simulink model "step_01_speed_measurement"  (R2021b)
settings: Solver=FixedStepAuto  StartTime=0.0  StopTime=1.5  FixedStep=1e-6  RelTol=1e-3
model workspace (MATLAB code in the model file):
  | %% DC motor parameteres
  | % High power w/ carbon brushes [3075]
  | % https://github.com/kpierzynski/MiniEmpathiaBot/blob/master/datasheets/POLOLU_N20_MOTOR.pdf
  | Vn = 6;          % [V]
  | Te_stall = 16;   % [kg*mm]
  | S_no_load = 330; % [rpm]
  | N_gear = 100.37; % [-]
  | 
  | La = 1e-4;       % [H]       -> ???
  | J = 1e-7;        % [kg*m^2]  -> ???
  | 
  | %% Incremental encoder parameteres
  | p_enc = 12;  % [pulses per revolution]
  | V_enc = 3.3; % [V]
  | 
  | %% Speed measurement algorithm parameteres
  | % method M sample time
  | Ts = 1e-3; % [s]
  | % Low-pass filter
  | % TODO
libraries: fl_lib x8, nesl_utility x7, spsEdgeDetectorLib x3, ee_lib x2, cstblocks x1, eeGeneralControl x1
settings Model: Creator=adria  LastModifiedBy=adria

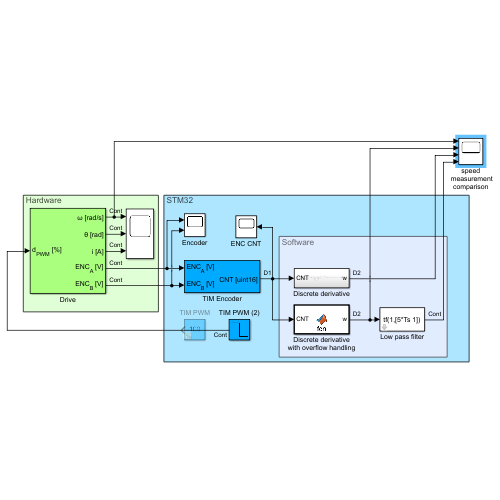
[thumbnail: Simulink's stored preview of the top-level diagram]
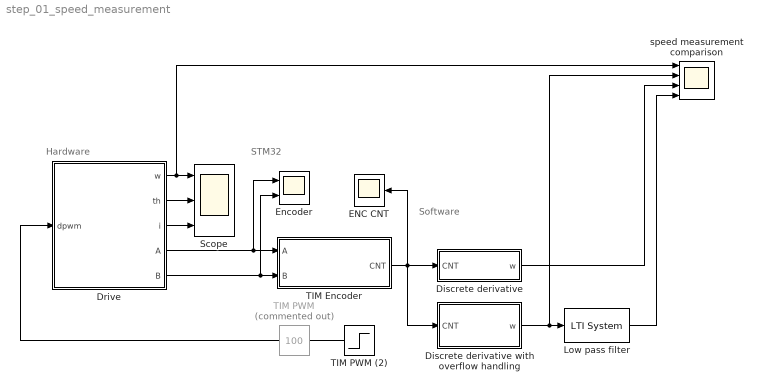
== system step_01_speed_measurement ==
  note: Software
  note: STM32
  note: Hardware
  Discrete derivative : Subsystem
  Discrete derivative with overflow handling : MATLAB Function  TreatAsAtomicUnit=on
  Drive : Subsystem
      mask Display:
      | port_label('input',1,'d_{PWM} [%]','texmode','on');
      | port_label('output',1,'\omega [rad/s]','texmode','on');
      | port_label('output',2,'\theta [rad]','texmode','on');
      | port_label('output',3,'i [A]','texmode','on');
      | port_label('output',4,'ENC_A [V]','texmode','on');
      | port_label('output',5,'ENC_B [V]','texmode','on');
  ENC CNT : Scope
  Encoder : Scope  NumInputPorts=2
  Low pass filter : cstblocks/LTI System  sys=tf(1,[5*Ts 1])  IC=[]
  Scope : Scope  NumInputPorts=3
  TIM Encoder : Subsystem
      mask Display:
      | port_label('input',1','ENC_A [V]','texmode','on');
      | port_label('input',2','ENC_B [V]','texmode','on');
      | port_label('output',1','CNT [uint16]','texmode','on');
  TIM PWM : Constant  Commented=on  Value=100
  TIM PWM (2) : Step  Time=0.5  Before=100  After=-100  SampleTime=0
  speed measurement comparison : Scope  NumInputPorts=4
  wires:
  TIM PWM (2)/1 -> Drive/1(dpwm)
  Drive/1(w) -> speed measurement comparison/1, Scope/1
  Drive/2(th) -> Scope/2
  Drive/3(i) -> Scope/3
  Drive/4(A) -> TIM Encoder/1(A), Encoder/1
  Drive/5(B) -> Encoder/2, TIM Encoder/2(B)
  TIM Encoder/1(CNT) -> Discrete derivative with overflow handling/1(CNT), Discrete derivative/1(CNT), ENC CNT/1
  Discrete derivative with overflow handling/1(w) -> speed measurement comparison/2, Low pass filter/1
  Low pass filter/1 -> speed measurement comparison/4
  Discrete derivative/1(w) -> speed measurement comparison/3

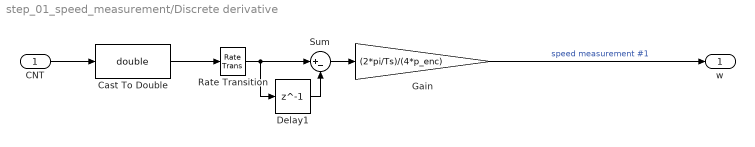
== system step_01_speed_measurement/Discrete derivative ==
  CNT : Inport
  Cast To Double : DataTypeConversion  OutDataTypeStr=double
  Delay1 : Delay  DelayLength=1  InitialCondition=60000  SampleTime=Ts
  Gain : Gain  Gain=(2*pi/Ts)/(4*p_enc)
  Rate Transition : RateTransition  OutPortSampleTime=Ts
  Sum : Sum  Inputs=|+-
  w : Outport  Unit=rad/s
  wires:
  Gain/1 -> w/1  "speed measurement #1"
  CNT/1 -> Cast To Double/1
  Sum/1 -> Gain/1
  Delay1/1 -> Sum/2
  Rate Transition/1 -> Delay1/1, Sum/1
  Cast To Double/1 -> Rate Transition/1

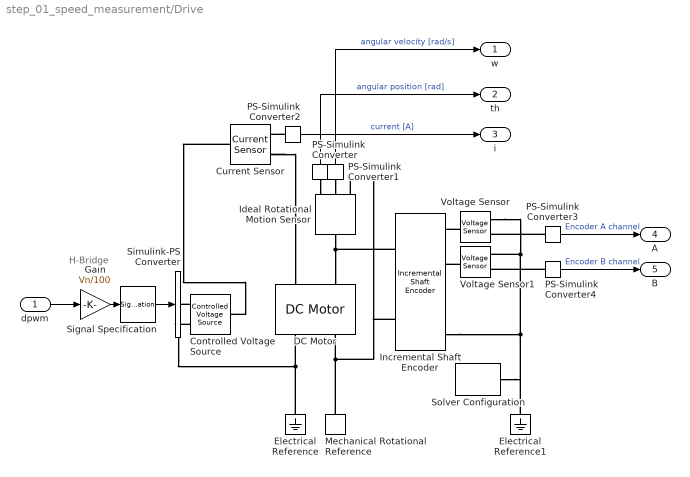
== system step_01_speed_measurement/Drive ==
  note: H-Bridge
  dpwm : Inport  Unit=1
  Controlled Voltage Source : fl_lib/Electrical/Electrical Sources/Controlled Voltage Source
  Current Sensor : fl_lib/Electrical/Electrical Sensors/Current Sensor
  DC Motor : ee_lib/Electromechanical/Brushed Motors/DC Motor  field_option=ee.enum.field_option.pm  Rf=100 Ohm  Lf=1 H  Laf=0.15 H  If0=0 A  parameterization=ee.enum.dcparam_option.torque_speed  Ra=Ra Ohm  La=La H  emf_or_torque=ee.enum.emf_or_torque.kv  Kv=2e-3 V/(rad/s)  Ki=6.876e-4 N*m/A  T_stall=Te_stall mN*m  w_max=S_no_load*N_gear rpm  w_rated=15000 rpm  P_rated=0.08 W  V_rated=Vn V  lam_param=ee.enum.lam_param.damping  i_noload=0 A  V_i_noload=1.5 V  J=J kg*m^2  lam=0 N*m/(rad/s)  speed0=0 rpm  enable_fault_armature=simscape.enum.onoff.off  rev_faulted=1 / 3  G_faulted_armature=1e-5 S  fault_trigger_armature=ee.enum.faults.faultTrigger.temporal  t_fault_armature=1 s  max_permissible_current_armature=inf A  t_fail_on_current_armature=1 s  enable_fault_field=simscape.enum.onoff.off  G_faulted_field=1e-5 S  fault_trigger_field=ee.enum.faults.faultTrigger.temporal  t_fault_field=1 s  max_permissible_current_field=inf A  t_fail_on_current_field=1 s  fault_action=simscape.enum.assert.action.none  alpha=3.93e-3 1/K  Tmeas=25 degC  thermal_mass=100 J/K  initial_temperature=25 degC
  Electrical Reference : fl_lib/Electrical/Electrical Elements/Electrical Reference
  Electrical Reference1 : fl_lib/Electrical/Electrical Elements/Electrical Reference
  Gain : Gain  Gain=Vn/100
  Ideal Rotational Motion Sensor : fl_lib/Mechanical/Mechanical Sensors/Ideal Rotational Motion Sensor  wrap_angle=simscape.enum.onoff.on  offset=0 rad
  Incremental Shaft Encoder : ee_lib/Sensors & Transducers/Incremental Shaft Encoder  NPulse=p_enc  Vm=V_enc V  angle0=0 deg
      settings: SourceProductBaseCode=PS  InternalSimscapePortConfiguration="{\"Bottom\":[],\"Left\":[{\"id\":\"R\",\"label\":\"R\",\"type\":\"foundation.mechanical.rotational.rotational\"},{\"id\":\"C\",\"label\":\"C\",\"type\":\"foundation.mechanical.rotational.rotational\"}],\"Right\":[{\"id\":\"A\",\"label\":\"A\",\"type\":\"foundation.electrical.electrical\"},{\"id\":\"B\",\"label\":\"B\",\"type\":\"foundation.electrical.electrical\"},{\"id\":\"Z\",\"label\":\"Z\",\"type\":\"foundation.electrical.electrical\"},{\"id\":\"GND\",\"label\":\"REF\",\"type\":\"foundation.electrical.electrical\"}],\"Top\":[]}"
  Mechanical Rotational Reference : fl_lib/Mechanical/Rotational Elements/Mechanical Rotational Reference
  PS-Simulink Converter{,1..4} (5 alike) : nesl_utility/PS-Simulink Converter  PhysicalDomain=network_engine_domain  SubClassName=ps_output  LeftPortType=input  RightPortType=output  PseudoPeriodic=off  Frequencies=[]  Unit=inherit  AffineConversion=off
      settings: SourceProductBaseCode=PW,SS
  Signal Specification : SignalSpecification  Unit=V
  Simulink-PS Converter : nesl_utility/Simulink-PS Converter  PhysicalDomain=network_engine_domain  SubClassName=ps_input  LeftPortType=input  RightPortType=output  PseudoPeriodic=off  Frequencies=[]  NoiseDistribution=none  NoiseParameters=[]  Unit=V  AffineConversion=off  FilteringAndDerivatives=provide  SimscapeFilterOrder=1  InputFilterTimeConstant=0.001  UdotUserProvided=0
      settings: SourceProductBaseCode=PW,SS
  Solver Configuration : nesl_utility/Solver Configuration  PhysicalDomain=network_engine_domain  SubClassName=solver  LeftPortType=input  RightPortType=generic  Tones=[]  Harmonics=[]  SimulateNoise=off  Profile=off  UseLocalSampling=off  EnableSwitchedLinearOptims=on  FrequencyDomain=off  UseCCode=off  RelTol=0.001  AbsTol=1e-06  MinStep=1e-09  ToWorkspace=off  RevertToSquareIcSolve=off  NumHomotopyIterations=100  PhasorMode=off  PhasorModeNumHarmonics=1  DoDC=off  ResidualTolerance=1e-09  UseLocalSolver=off  LocalSolverChoice=NE_BACKWARD_EULER_ADVANCER  LocalSolverSampleTime=0.001  DoFixedCost=off  MaxNonlinIter=3  MaxModeIter=2  ComputeImpulses=off  ImpulseIterations=2  LinearAlgebra=auto  EquationFormulation=NE_TIME_EF  DelaysMemoryBudget=1024  AutomaticFiltering=on  FilteringTimeConstant=0.001  PartitionStorageMethod=AS_NEEDED  PartitionMemoryBudget=1024  PartitionMethod=ROBUST
      settings: SourceProductBaseCode=PW,SS
  Voltage Sensor : fl_lib/Electrical/Electrical Sensors/Voltage Sensor
  Voltage Sensor1 : fl_lib/Electrical/Electrical Sensors/Voltage Sensor
  w : Outport  Unit=rad/s
  th : Outport  Port=2  Unit=rad
  i : Outport  Port=3  Unit=A
  A : Outport  Port=4  Unit=V
  B : Outport  Port=5  Unit=V
  wires:
  PS-Simulink Converter2/1 -> i/1  "current [A]"
  PS-Simulink Converter/1 -> th/1  "angular position [rad]"
  PS-Simulink Converter3/1 -> A/1  "Encoder A channel"
  dpwm/1 -> Gain/1
  PS-Simulink Converter4/1 -> B/1  "Encoder B channel"
  PS-Simulink Converter1/1 -> w/1  "angular velocity [rad/s]"
  Gain/1 -> Signal Specification/1
  Signal Specification/1 -> Simulink-PS Converter/1
  connections:
  Ideal Rotational Motion Sensor/RConn1 -- Incremental Shaft Encoder/LConn2 -- DC Motor/RConn2 -- Mechanical Rotational Reference/LConn1
  Controlled Voltage Source/RConn2 -- DC Motor/RConn1 -- Electrical Reference/LConn1
  Solver Configuration/RConn1 -- Electrical Reference1/LConn1 -- Incremental Shaft Encoder/RConn4 -- Voltage Sensor/RConn2 -- Voltage Sensor1/RConn2
  Incremental Shaft Encoder/LConn1 -- DC Motor/LConn2 -- Ideal Rotational Motion Sensor/LConn1
  Voltage Sensor/LConn1 -- Incremental Shaft Encoder/RConn1
  PS-Simulink Converter3/LConn1 -- Voltage Sensor/RConn1
  Voltage Sensor1/LConn1 -- Incremental Shaft Encoder/RConn2
  Current Sensor/LConn1 -- Controlled Voltage Source/LConn1
  PS-Simulink Converter1/LConn1 -- Ideal Rotational Motion Sensor/RConn2
  PS-Simulink Converter/LConn1 -- Ideal Rotational Motion Sensor/RConn3
  Controlled Voltage Source/RConn1 -- Simulink-PS Converter/RConn1
  PS-Simulink Converter2/LConn1 -- Current Sensor/RConn1
  PS-Simulink Converter4/LConn1 -- Voltage Sensor1/RConn1
  Current Sensor/RConn2 -- DC Motor/LConn1

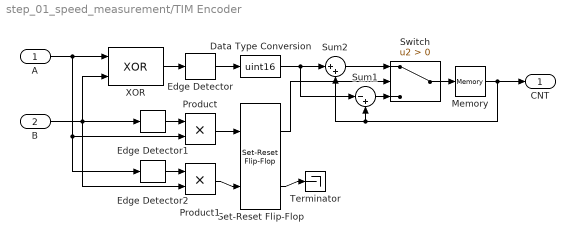
== system step_01_speed_measurement/TIM Encoder ==
  A : Inport
  B : Inport  Port=2
  Data Type Conversion : DataTypeConversion  OutDataTypeStr=uint16
  Edge Detector : spsEdgeDetectorLib/Edge Detector  model=Either  ic=0  Ts=0
      settings: SourceProductBaseCode=PS
  Edge Detector1 : spsEdgeDetectorLib/Edge Detector  model=Rising  ic=0  Ts=0
      settings: SourceProductBaseCode=PS
  Edge Detector2 : spsEdgeDetectorLib/Edge Detector  model=Rising  ic=0  Ts=0
      settings: SourceProductBaseCode=PS
  Memory : Memory  InitialCondition=60000
  Product : Product
  Product1 : Product
  Set-Reset Flip-Flop : eeGeneralControl/Set-Reset Flip-Flop  LabelModeActiveChoice=Discrete  UndefState=Set  Q0=1  Ts=-1
      settings: SourceProductBaseCode=PS
  Sum1 : Sum  Inputs=|-+
  Sum2 : Sum  Inputs=|++
  Switch : Switch  Criteria=u2 > Threshold
  Terminator : Terminator
  XOR : Logic  Operator=XOR  IconShape=distinctive  AllPortsSameDT=off  OutDataTypeStr=boolean
  CNT : Outport  OutDataTypeStr=uint16
  wires:
  Set-Reset Flip-Flop/2 -> Terminator/1
  Product/1 -> Set-Reset Flip-Flop/1
  Data Type Conversion/1 -> Sum1/1, Sum2/1
  Product1/1 -> Set-Reset Flip-Flop/2
  Set-Reset Flip-Flop/1 -> Switch/2
  Edge Detector/1 -> Data Type Conversion/1
  B/1 -> XOR/2, Product1/2, Edge Detector1/1
  XOR/1 -> Edge Detector/1
  Switch/1 -> Memory/1
  A/1 -> Edge Detector2/1, Product/2, XOR/1
  Edge Detector1/1 -> Product/1
  Sum2/1 -> Switch/1
  Memory/1 -> CNT/1, Sum1/2, Sum2/2
  Edge Detector2/1 -> Product1/1
  Sum1/1 -> Switch/3

== matlab function step_01_speed_measurement/Discrete derivative with overflow handling ==
  settings: updateMethod=DISCRETE  sampleTime=Ts
  data: CNT input; w output
function w = fcn(CNT)
%% Speed measurement algorithm parameteres
p_enc = 12; % [ppr]
Ts = 1e-3;  % [s] 

%% Local variables
persistent CNT_Prev

if isempty(CNT_Prev)
    CNT_Prev = 60000;
end
CNT_DiffMax = 2^16; % [uint16]
CNT = double(CNT);

%% Measurement logic

% Compute difference between current and previous counter value
CNT_Diff = CNT - CNT_Prev;

% Handle integer overflow
if abs(CNT_Diff) > CNT_DiffMax/2
    CNT_Diff = CNT + sign(CNT_Diff)*CNT_Prev - sign(CNT_Diff)*CNT_DiffMax;
end

% Save counter value for next iteration
CNT_Prev = CNT;

% Scale result to rad/s
w = ((2*pi/Ts)/(4*p_enc)) * CNT_Diff;
